simulink model "P2_simulink_1"  (R2017a)
settings: Solver=VariableStepAuto  StartTime=0.0  StopTime=10.0  RelTol=1e-3  EnableMultiTasking=on
values from neighbouring files (symbols this model uses):
  b = 0.5    [P2_datos.m]
  g = 9.8    [P2_datos.m]
  k = 2    [P2_datos.m]
  L = 0.01    [P2_datos.m]
  M = 0.2    [P2_datos.m]
  R = 20    [P2_datos.m]
settings Model: Creator=Administrador  LastModifiedBy=feder
settings DataIOCC: LimitDataPoints=on  SaveFormat=Array
settings OptimizationCC: LifeSpan=inf
settings DebuggingCC: SolverPrmCheckMsg=warning  SFUnexpectedBacktrackingDiag=warning  SFNoUnconditionalDefaultTransitionDiag=warning  SFExecutionAtInitializationDiag=none
settings HardwareCC: ProdBitPerPointer=32  ProdBitPerSizeT=32  ProdBitPerPtrDiffT=32  ProdLargestAtomicFloat=None  ProdIntDivRoundTo=Undefined  ProdEndianess=Unspecified  ProdWordSize=32  ProdHWDeviceType=32-bit Generic
settings ModelReferenceCC: PropagateSignalLabelsOutOfModel=off
settings GRTTargetCC: TargetLangStandard=C89/C90 (ANSI)  GeneratePreprocessorConditionals=Disable all
settings ConfigComp: CovMetricSettings=dw  CovHtmlReporting=on  CovSaveCumulativeToWorkspaceVar=on  CovSaveSingleToWorkspaceVar=on  CovExternalEMLEnable=off  CovSFcnEnable=off

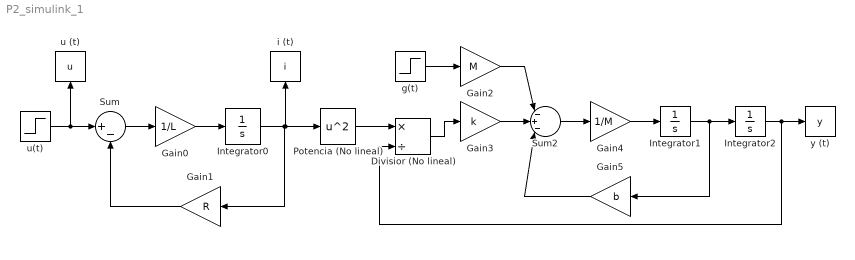
== system P2_simulink_1 ==
  " i (t)" : ToWorkspace  VariableName=i  SaveFormat=Timeseries  SampleTime=-1
  " u (t)" : ToWorkspace  VariableName=u  SaveFormat=Timeseries  SampleTime=-1
  Divisior (No lineal) : Product  Inputs=*/
  Gain0 : Gain  Gain=1/L
  Gain1 : Gain  Gain=R
  Gain2 : Gain  Gain=M
  Gain3 : Gain  Gain=k
  Gain4 : Gain  Gain=1/M
  Gain5 : Gain  Gain=b
  Integrator0 : Integrator  InitialCondition=0.5
  Integrator1 : Integrator
  Integrator2 : Integrator  InitialCondition=0.2551
  Potencia (No lineal) : Math  Operator=square  SaturateOnIntegerOverflow=on
  Sum : Sum  Inputs=|+-
  Sum2 : Sum  Inputs=|-+-|
  g(t) : Step  Time=0  After=g  SampleTime=0
  u(t) : Step  Time=0  Before=10  After=12  SampleTime=0
  y (t) : ToWorkspace  VariableName=y  SaveFormat=Timeseries  SampleTime=-1
  wires:
  Sum/1 -> Gain0/1
  Gain0/1 -> Integrator0/1
  Integrator0/1 -> Potencia (No lineal)/1, " i (t)"/1, Gain1/1
  Gain1/1 -> Sum/2
  Integrator1/1 -> Integrator2/1, Gain5/1
  Integrator2/1 -> y (t)/1, Divisior (No lineal)/2
  Gain4/1 -> Integrator1/1
  u(t)/1 -> " u (t)"/1, Sum/1
  g(t)/1 -> Gain2/1
  Gain2/1 -> Sum2/1
  Gain5/1 -> Sum2/3
  Sum2/1 -> Gain4/1
  Potencia (No lineal)/1 -> Divisior (No lineal)/1
  Divisior (No lineal)/1 -> Gain3/1
  Gain3/1 -> Sum2/2
